simulink model "stp2_1"  (R2016b)
settings: Solver=VariableStepAuto  StartTime=0.0  StopTime=10.0  RelTol=1e-3
undefined symbols (not defined in the file): Ad, Cd
settings Model: Creator=arq  LastModifiedBy=arq

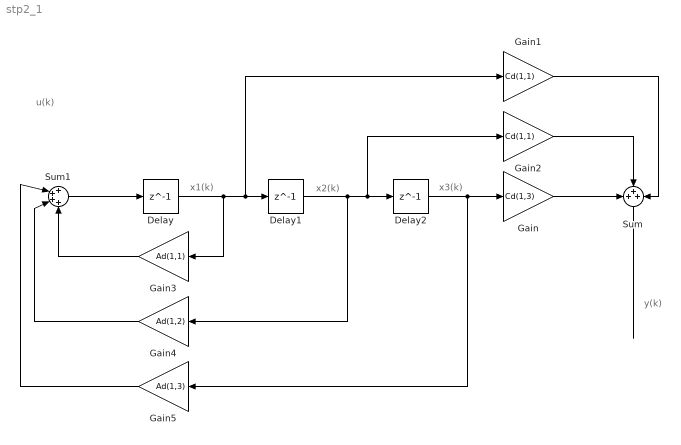
== system stp2_1 ==
  note: u(k)
  note: x3(k)
  note: x2(k)
  note: x1(k)
  note: y(k)
  Delay : Delay  DelayLength=1  InitialCondition=0
  Delay1 : Delay  DelayLength=1  InitialCondition=0
  Delay2 : Delay  DelayLength=1  InitialCondition=0
  Gain : Gain  Gain=Cd(1,3)
  Gain1 : Gain  Gain=Cd(1,1)
  Gain2 : Gain  Gain=Cd(1,1)
  Gain3 : Gain  Gain=Ad(1,1)
  Gain4 : Gain  Gain=Ad(1,2)
  Gain5 : Gain  Gain=Ad(1,3)
  Sum : Sum  Inputs=3
  Sum1 : Sum  Inputs=4
  wires:
  Delay/1 -> Gain3/1, Gain1/1, Delay1/1
  Delay1/1 -> Gain4/1, Gain2/1, Delay2/1
  Delay2/1 -> Gain5/1, Gain/1
  Gain/1 -> Sum/1
  Gain2/1 -> Sum/2
  Gain1/1 -> Sum/3
  Sum/1 -> ?
  Sum1/1 -> Delay/1
  ? -> Sum1/1
  Gain3/1 -> Sum1/4
  Gain4/1 -> Sum1/3
  Gain5/1 -> Sum1/2
